simulink model "PSS2B_block"  (R2020a)
settings: Solver=FixedStepAuto  StartTime=0.0  StopTime=16.5  FixedStep=0.005  RelTol=1e-3
values from neighbouring files (symbols this model uses):
  K_S1 = 5.028    [Nonlinear_simulation_compare.m]    (also in essai5JUne_initMostar.mat = 2.0489)
  K_S2 = 0.3542    [Nonlinear_simulation_compare.m]    (also in essai5JUne_initMostar.mat = 5.02712)
  K_S3 = 1.0198    [Nonlinear_simulation_compare.m]    (also in essai5JUne_initMostar.mat = 0.44074)
  T_1 = 0.1103    [Nonlinear_simulation_compare.m]    (also in essai5JUne_initMostar.mat = 0.208823)
  T_10 = 0.01    [Nonlinear_simulation_compare.m]    (also in essai5JUne_initMostar.mat = 0.009203)
  T_11 = 0.01    [Nonlinear_simulation_compare.m]    (also in essai5JUne_initMostar.mat = 0.013378)
  T_2 = 0.0404    [Nonlinear_simulation_compare.m]    (also in essai5JUne_initMostar.mat = 0.045679)
  T_3 = 0.3147    [Nonlinear_simulation_compare.m]    (also in essai5JUne_initMostar.mat = 0.38894)
  T_4 = 0.1162    [Nonlinear_simulation_compare.m]    (also in essai5JUne_initMostar.mat = 0.1209067)
  T_6 = 0.0027    [Nonlinear_simulation_compare.m]    (also in essai5JUne_initMostar.mat = 0.0105388)
  T_7 = 2.0811    [Nonlinear_simulation_compare.m]    (also in essai5JUne_initMostar.mat = 1.0215)
  T_8 = -0.0009    [Nonlinear_simulation_compare.m]    (also in essai5JUne_initMostar.mat = 0.33863)
  T_9 = 0.101    [Nonlinear_simulation_compare.m]    (also in essai5JUne_initMostar.mat = 0.14362)
  T_w1 = 2.0118    [Nonlinear_simulation_compare.m]    (also in essai5JUne_initMostar.mat = 1.9675)
  T_w2 = 1.9506    [Nonlinear_simulation_compare.m]    (also in essai5JUne_initMostar.mat = 2.137)
  T_w3 = 1.939    [Nonlinear_simulation_compare.m]    (also in essai5JUne_initMostar.mat = 2.1786)
  T_w4 = 1.9782    [Nonlinear_simulation_compare.m]    (also in essai5JUne_initMostar.mat = 2.002)
  V_S1MAX = 0.8    [Nonlinear_simulation_compare.m]    (also in essai5JUne_initMostar.mat)
  V_S1MIN = -0.8    [Nonlinear_simulation_compare.m]    (also in essai5JUne_initMostar.mat)
  V_S2MAX = 1.25    [Nonlinear_simulation_compare.m]    (also in essai5JUne_initMostar.mat)
  V_S2MIN = -1.25    [Nonlinear_simulation_compare.m]    (also in essai5JUne_initMostar.mat)
  V_STMAX = 0.1    [Nonlinear_simulation_compare.m]    (also in essai5JUne_initMostar.mat)
  V_STMIN = -0.1    [Nonlinear_simulation_compare.m]    (also in essai5JUne_initMostar.mat)
settings Model: Creator=meagh  LastModifiedBy=meagh

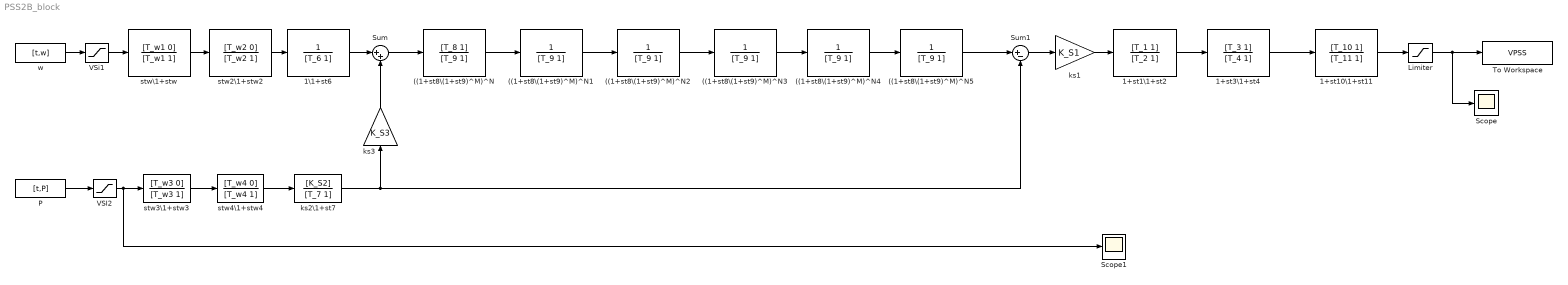
== system PSS2B_block ==
  ((1+st8\(1+st9)^M)^N : TransferFcn  Numerator=[T_8 1]  Denominator=[T_9 1]
  ((1+st8\(1+st9)^M)^N{1..5} (5 alike) : TransferFcn  Denominator=[T_9 1]
  1+st10\1+st11 : TransferFcn  Numerator=[T_10 1]  Denominator=[T_11 1]
  1+st1\1+st2 : TransferFcn  Numerator=[T_1 1]  Denominator=[T_2 1]
  1+st3\1+st4 : TransferFcn  Numerator=[T_3 1]  Denominator=[T_4 1]
  1\1+st6 : TransferFcn  Denominator=[T_6 1]
  "Limiter " : Saturate  UpperLimit=V_STMAX  LowerLimit=V_STMIN
  P : FromWorkspace  VariableName=[t,P]
  Scope : Scope
  Scope1 : Scope
  Sum : Sum  Inputs=|++
  Sum1 : Sum  Inputs=|+-
  To Workspace : ToWorkspace  VariableName=VPSS  SaveFormat=Timeseries  SampleTime=0.005
  VSI2 : Saturate  UpperLimit=V_S2MAX  LowerLimit=V_S2MIN
  VSi1 : Saturate  UpperLimit=V_S1MAX  LowerLimit=V_S1MIN
  ks1 : Gain  Gain=K_S1  SaturateOnIntegerOverflow=on  OutDataTypeStr=Inherit: Same as input  ParamDataTypeStr=Inherit: Same as input
  ks2\1+st7 : TransferFcn  Numerator=[K_S2]  Denominator=[T_7 1]
  ks3 : Gain  Gain=K_S3  SaturateOnIntegerOverflow=on  OutDataTypeStr=Inherit: Same as input  ParamDataTypeStr=Inherit: Same as input
  stw2\1+stw2 : TransferFcn  Numerator=[T_w2 0]  Denominator=[T_w2 1]
  stw3\1+stw3 : TransferFcn  Numerator=[T_w3 0]  Denominator=[T_w3 1]
  stw4\1+stw4 : TransferFcn  Numerator=[T_w4 0]  Denominator=[T_w4 1]
  stw\1+stw : TransferFcn  Numerator=[T_w1 0]  Denominator=[T_w1 1]
  w : FromWorkspace  VariableName=[t,w]
  wires:
  ks1/1 -> 1+st1\1+st2/1
  1+st3\1+st4/1 -> 1+st10\1+st11/1
  stw3\1+stw3/1 -> stw4\1+stw4/1
  ks2\1+st7/1 -> Sum1/2, ks3/1
  stw2\1+stw2/1 -> 1\1+st6/1
  ks3/1 -> Sum/2
  ((1+st8\(1+st9)^M)^N/1 -> ((1+st8\(1+st9)^M)^N1/1
  Sum1/1 -> ks1/1
  stw4\1+stw4/1 -> ks2\1+st7/1
  1\1+st6/1 -> Sum/1
  stw\1+stw/1 -> stw2\1+stw2/1
  1+st1\1+st2/1 -> 1+st3\1+st4/1
  P/1 -> VSI2/1
  VSI2/1 -> Scope1/1, stw3\1+stw3/1
  w/1 -> VSi1/1
  1+st10\1+st11/1 -> "Limiter "/1
  ((1+st8\(1+st9)^M)^N1/1 -> ((1+st8\(1+st9)^M)^N2/1
  ((1+st8\(1+st9)^M)^N2/1 -> ((1+st8\(1+st9)^M)^N3/1
  ((1+st8\(1+st9)^M)^N3/1 -> ((1+st8\(1+st9)^M)^N4/1
  ((1+st8\(1+st9)^M)^N4/1 -> ((1+st8\(1+st9)^M)^N5/1
  ((1+st8\(1+st9)^M)^N5/1 -> Sum1/1
  "Limiter "/1 -> Scope/1, To Workspace/1
  VSi1/1 -> stw\1+stw/1
  Sum/1 -> ((1+st8\(1+st9)^M)^N/1
